simulink model "dynamics_lab2"  (Simulink 7.9)
settings: Solver=ode1  StartTime=0.0  StopTime=1000  FixedStep=0.1  RelTol=1e-3
InitFcn:
  | clear all;close all;clc;warning off all;
  | 
  | 
  | % Simulation run parameters
  | Rate=34.3; DeltaT=1/Rate;
  | 
  | % Maneuver Parameters
  | roll=0; pitch=0; yaw=30; roll=roll*pi/180; pitch=pitch*pi/180; yaw=yaw*pi/180;
  | SlewTime=5; SACengage=0;
  | Re=6371.2e3;mu=398601.2e9; %earth radius and universal gravitation constant
  | 
  | %Spacecraft orbit
  | h=180e3; %orbit altitude in meters
  | R=Re+h; %orbit radius from center of earth
  | we=0.000072921158553; %earth's angular velocity rad/solar sec(Vallado)
  | wo=sqrt(mu/(Re+h)^3);
  | 
  | 
  | %Spacecraft Inertia conditions
  | Ix=119.1259; Iy=150.6615; Iz=106.0288;
  | Ixy=0; Iyz=0; Ixz=0;
  | Imo=[Ix Ixy Ixz;
  | Ixy Iy Iyz;
  | Ixz Iyz Iz]; %Moment of inertia matrix
  | Iinv=inv(Imo); %Moment of inertia inverse goes in dynamics block
  | 
  | %Spacecraft initial Euler state angles and rates
  | phio=4*pi/180;thetao=-4*pi/180;psio=4*pi/180; %Initial Euler Angles
  | phidoto=0.15*pi/180;thetadoto=0.15*pi/180;psidoto=0.15*pi/180; %Initial Euler Rates
  | alfinit=[phio thetao psio];
  | winit=[phidoto thetadoto psidoto];
  | 
  | %Calculation of initial quaternion (qo) and angular momentum (Ho)
  | s1=sin(phio/2);s2=sin(thetao/2);s3=sin(psio/2);c1=cos(phio/2);c2=cos(thetao/2);c3=cos(psio/2);
  | q1o=s1*c2*c3-c1*s2*s3;
  | q2o=c1*s2*c3+s1*c2*s3; %Wie pg. 321
  | q3o=c1*c2*s3-s1*s2*c3;
  | q4o=c1*c2*c3+s1*s2*s3;
  | S1=sin(phio);S2=sin(thetao);S3=sin(psio);C1=cos(phio);C2=cos(thetao);C3=cos(psio);
  | wxo=phidoto-psidoto*S2-wo*S3*C2;
  | wyo=thetadoto*C1+psidoto*C2*S1-wo*(C3*C1+S3*S2*S1);
  | wzo=psidoto*C2*C1-thetadoto*S1-wo*(S3*S2*C1-C3*S1);
  | qo=[q1o q2o q3o q4o];
  | Ho=Imo*[wxo wyo wzo]';
  | 
  | x=[4 4 4 2 2 2];%xmax
  | u=[2.1 2.1 2.1];%umax
  | J=[Ix Iy Iz];  % J of the system
  | 
  | Jinv=J';
  | 
  | hom=0.001; %rad/s
  | N=0;
  | %Linear quadratic Regulator
  | A=[0,0,0,1,0,0;0,0,0,0,1,0;0,0,0,0,0,1;4*((J(3)-J(2))/J(1))*(hom^2),0,0,0,0,((J(3)+J(1)-J(2))/J(1))*hom;0,3*((J(3)-J(1))/J(2))*(hom^2),0,0,0,0;0,0,((J(1)-J(2))/J(3))*(hom^2),(((J(2)-J(1)-J(3))/J(3))*hom),0,0];
  | B=[0,0,0;0,0,0;0,0,0;1/J(1),0,0;0,1/J(2),0;0,0,1/J(3)];
  | Q=[1/(x(1)^2),0,0,0,0,0;0,1/(x(2)^2),0,0,0,0;0,0,1/(x(3)^2),0,0,0;0,0,0,1/(x(4)^2),0,0;0,0,0,0,1/(x(5)^2),0;0,0,0,0,0,1/(x(6)^2)];
  | R=[100/(u(1)^2),0,0;0,100/(u(2)^2),0;0,0,100/(u(3)^2)];
  | 
  |  K=lqr(A,B,Q,R,N);
  | 
  | %State Estimator
  | 
  | %C=[1,0,0,0,0,0;0,1,0,0,0,0;0,0,1,0,0,0;0,0,0,0,0,0;0,0,0,0,0,0;0,0,0,0,0,0];
  | 
  | C=eye(6,6);
  | Q1=eye(6,6);
  | R1=eye(6,6);
  | 
  | L=[lqr(A',C',Q1,R1)]';
libraries: aerospace x2, simulink x1
settings Model: Creator=bleonard  LastModifiedBy=Alex
settings OptimizationCC: InitFltsAndDblsToZero=on
settings DebuggingCC: SaveWithParameterizedLinksMsg=none  MultiTaskCondExecSysMsg=none  StrictBusMsg=None
settings RTWCC: IncludeERTFirstTime=on
settings GRTTargetCC: CombineOutputUpdateFcns=off  GRTInterface=on

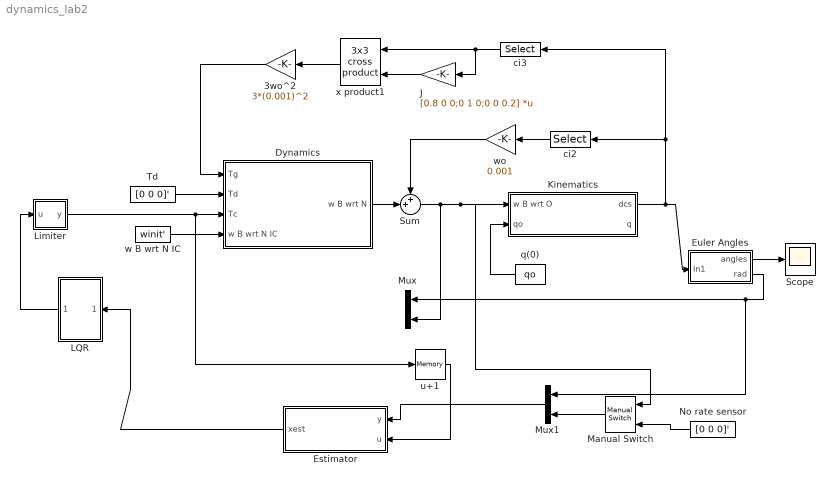
== system dynamics_lab2 ==
  3wo^2 : Gain  Gain=3*(0.001)^2
  Dynamics : Subsystem
  Estimator : Subsystem
  Euler Angles : Subsystem
  J : Gain  Gain=[0.8 0 0;0 1 0;0 0 0.2]  Multiplication=Matrix(K*u)  SaturateOnIntegerOverflow=on  OutDataTypeStr=Inherit: Same as input  ParamDataTypeStr=Inherit: Same as input
  Kinematics : Subsystem
  LQR : Subsystem
  Limiter : MATLAB Function  TreatAsAtomicUnit=on
  Manual Switch : simulink/Signal Routing/Manual Switch  sw=0  action=0  varsize=off
  Mux : Mux  Inputs=2
  Mux1 : Mux  Inputs=2
  No rate sensor : Constant  Value=[0 0 0]'
  Scope : Scope
  Sum : Sum  Inputs=++|
  Td : Constant  Value=[0 0 0]'
  ci2 : Selector  InputPortWidth=9  IndexOptions=Index vector (dialog)  Indices=[4 5 6]  OutputSizes=1
  ci3 : Selector  InputPortWidth=9  IndexOptions=Index vector (dialog)  Indices=[7 8 9]  OutputSizes=1
  q(0) : Constant  Value=qo
  u+1 : Memory  X0=[0 0 0]  InheritSampleTime=on
  w B wrt N IC : Constant  Value=winit'
  wo : Gain  Gain=0.001
  x product1 : aerospace/Axes Transformations/3x3 cross product
  wires:
  Td/1 -> Dynamics/2(Td)
  Dynamics/1(w B wrt N) -> Sum/2
  Sum/1 -> Mux/2, Kinematics/1(w B wrt O), Manual Switch/1
  Kinematics/1(dcs) -> ci2/1, ci3/1, Euler Angles/1(In1)
  ci2/1 -> wo/1
  wo/1 -> Sum/1
  ci3/1 -> J/1, x product1/1
  x product1/1 -> 3wo^2/1
  3wo^2/1 -> Dynamics/1(Tg)
  J/1 -> x product1/2
  w B wrt N IC/1 -> Dynamics/4(w B wrt N IC)
  Euler Angles/2(rad) -> Mux/1, Mux1/1
  LQR/1(Out1) -> Limiter/1(u)
  q(0)/1 -> Kinematics/2(qo)
  Euler Angles/1(angles) -> Scope/1
  Limiter/1(y) -> Dynamics/3(Tc), u+1/1
  Estimator/1(xest) -> LQR/1(In1)
  u+1/1 -> Estimator/2(u)
  Mux1/1 -> Estimator/1(y)
  Manual Switch/1 -> Mux1/2
  No rate sensor/1 -> Manual Switch/2

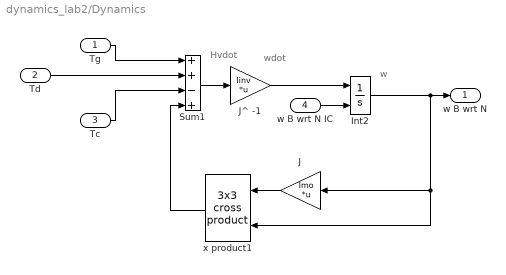
== system dynamics_lab2/Dynamics ==
  note: wdot
  note: Hvdot
  note: w
  Tg : Inport
  Td : Inport  Port=2
  Tc : Inport  Port=3
  w B wrt N IC : Inport  Port=4
  "   J^ -1" : Gain  Gain=Iinv  Multiplication=Matrix(K*u)  SaturateOnIntegerOverflow=on  OutDataTypeStr=Inherit: Same as input  ParamDataTypeStr=Inherit: Same as input
  Int2 : Integrator  InitialConditionSource=external  InitialCondition="[0  -0.001  0]'"
  J : Gain  Gain=Imo  Multiplication=Matrix(K*u)  SaturateOnIntegerOverflow=on  OutDataTypeStr=Inherit: Same as input  ParamDataTypeStr=Inherit: Same as input
  Sum1 : Sum  Inputs=++-+  SaturateOnIntegerOverflow=on  InputSameDT=on  OutDataTypeStr=Inherit: Same as first input
  x product1 : aerospace/Axes Transformations/3x3 cross product
  w B wrt N : Outport
  wires:
  Sum1/1 -> "   J^ -1"/1
  Int2/1 -> J/1, x product1/2, w B wrt N/1
  x product1/1 -> Sum1/4
  "   J^ -1"/1 -> Int2/1
  J/1 -> x product1/1
  Tg/1 -> Sum1/1
  Td/1 -> Sum1/2
  Tc/1 -> Sum1/3
  w B wrt N IC/1 -> Int2/2

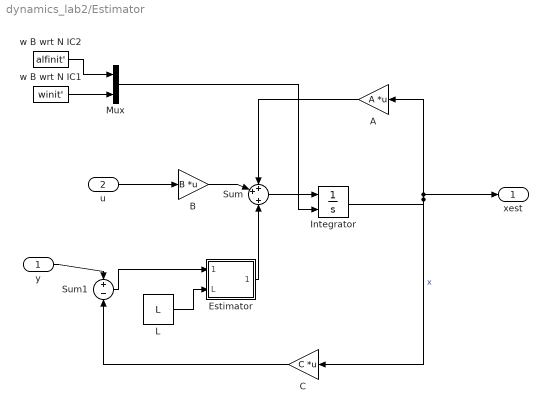
== system dynamics_lab2/Estimator ==
  y : Inport
  u : Inport  Port=2
  A : Gain  Gain=A  Multiplication=Matrix(K*u) (u vector)
  B : Gain  Gain=B  Multiplication=Matrix(K*u) (u vector)
  C : Gain  Gain=C  Multiplication=Matrix(K*u) (u vector)
  Estimator : MATLAB Function  TreatAsAtomicUnit=on
  Integrator : Integrator  InitialConditionSource=external
  L : Constant  Value=L
  Mux : Mux  Inputs=2
  Sum : Sum  Inputs=++|+
  Sum1 : Sum  Inputs=+-
  w B wrt N IC1 : Constant  Value=winit'
  w B wrt N IC2 : Constant  Value=alfinit'
  xest : Outport
  wires:
  u/1 -> B/1
  Sum/1 -> Integrator/1
  Integrator/1 -> A/1, xest/1, C/1  "x"
  B/1 -> Sum/2
  A/1 -> Sum/1
  y/1 -> Sum1/1
  C/1 -> Sum1/2
  Sum1/1 -> Estimator/1(y_est)
  Estimator/1(x_est) -> Sum/3
  L/1 -> Estimator/2(L)
  w B wrt N IC2/1 -> Mux/1
  w B wrt N IC1/1 -> Mux/2
  Mux/1 -> Integrator/2

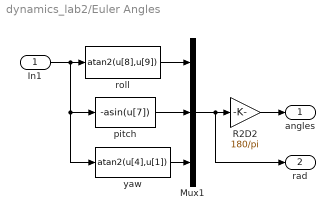
== system dynamics_lab2/Euler Angles ==
  In1 : Inport
  Mux1 : Mux  Inputs=3
  R2D2 : Gain  Gain=180/pi  SampleTime=0.1
  pitch : Fcn  Expr=-asin(u[7])
  roll : Fcn  Expr=atan2(u[8],u[9])
  yaw : Fcn  Expr=atan2(u[4],u[1])
  angles : Outport
  rad : Outport  Port=2
  wires:
  roll/1 -> Mux1/1
  yaw/1 -> Mux1/3
  pitch/1 -> Mux1/2
  Mux1/1 -> rad/1, R2D2/1
  In1/1 -> roll/1, pitch/1, yaw/1
  R2D2/1 -> angles/1

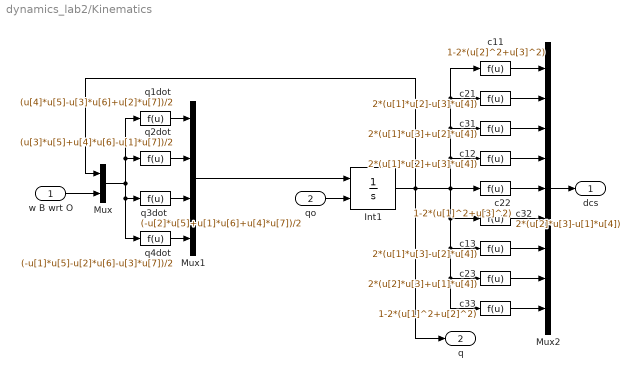
== system dynamics_lab2/Kinematics ==
  w B wrt O : Inport
  qo : Inport  Port=2
  Int1 : Integrator  InitialConditionSource=external  InitialCondition=[0 0 -0.1]'
  Mux : Mux  Inputs=2
  Mux1 : Mux
  Mux2 : Mux  Inputs=9
  c11 : Fcn  Expr=1-2*(u[2]^2+u[3]^2)
  c12 : Fcn  Expr=2*(u[1]*u[2]+u[3]*u[4])
  c13 : Fcn  Expr=2*(u[1]*u[3]-u[2]*u[4])
  c21 : Fcn  Expr=2*(u[1]*u[2]-u[3]*u[4])
  c22 : Fcn  Expr=1-2*(u[1]^2+u[3]^2)
  c23 : Fcn  Expr=2*(u[2]*u[3]+u[1]*u[4])
  c31 : Fcn  Expr=2*(u[1]*u[3]+u[2]*u[4])
  c32 : Fcn  Expr=2*(u[2]*u[3]-u[1]*u[4])
  c33 : Fcn  Expr=1-2*(u[1]^2+u[2]^2)
  q1dot : Fcn  Expr=(u[4]*u[5]-u[3]*u[6]+u[2]*u[7])/2
  q2dot : Fcn  Expr=(u[3]*u[5]+u[4]*u[6]-u[1]*u[7])/2
  q3dot : Fcn  Expr=(-u[2]*u[5]+u[1]*u[6]+u[4]*u[7])/2
  q4dot : Fcn  Expr=(-u[1]*u[5]-u[2]*u[6]-u[3]*u[7])/2
  dcs : Outport
  q : Outport  Port=2
  wires:
  Mux/1 -> q4dot/1, q3dot/1, q1dot/1, q2dot/1
  q1dot/1 -> Mux1/1
  q2dot/1 -> Mux1/2
  q3dot/1 -> Mux1/3
  q4dot/1 -> Mux1/4
  Int1/1 -> Mux/1, c22/1, c11/1, c21/1, c31/1, c12/1, c32/1, c13/1, c33/1, c23/1, q/1
  c11/1 -> Mux2/1
  c22/1 -> Mux2/5
  c33/1 -> Mux2/9
  c21/1 -> Mux2/2
  c31/1 -> Mux2/3
  c12/1 -> Mux2/4
  c32/1 -> Mux2/6
  c13/1 -> Mux2/7
  c23/1 -> Mux2/8
  Mux1/1 -> Int1/1
  w B wrt O/1 -> Mux/2
  Mux2/1 -> dcs/1
  qo/1 -> Int1/2

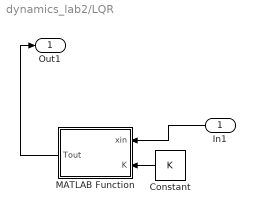
== system dynamics_lab2/LQR ==
  In1 : Inport
  Constant : Constant  Value=K
  MATLAB Function : MATLAB Function  TreatAsAtomicUnit=on
  Out1 : Outport
  wires:
  Constant/1 -> MATLAB Function/2(K)
  MATLAB Function/1(Tout) -> Out1/1
  In1/1 -> MATLAB Function/1(xin)

== matlab function Limiter ==
  data: u input double; y output double
function y = fcn(u)
%#codegen



if u(1) > 2.1
    
    y1=2.1;
else
    y1=u(1);
end

if u(2) > 2.1
    
    y2=2.1;
else
    y2=u(2);
end

if u(3) > 2.1
    
    y3=2.1;
else
    y3=u(3);
end


y=[y1 y2 y3]';

== matlab function LQR/MATLAB Function ==
  data: xin input double; Tout output double; K input double
function Tout = fcn(xin,K)
%#codegen



Tout = K*xin;

== matlab function Estimator/Estimator ==
  data: y_est input double; x_est output double; L input double
function x_est = fcn(y_est,L)
%#codegen



x_est=L*y_est;
